simulink model "sensorExpoler_Lab1_4"  (R2026a)
settings: Solver=FixedStepDiscrete  StopTime=inf  FixedStep=0.001
undefined symbols (not defined in the file or in its folder): Blocking, Non
libraries: amg_usbconverter_n_connect_lib x2
settings Model: Creator=pboon  LastModifiedBy=supha

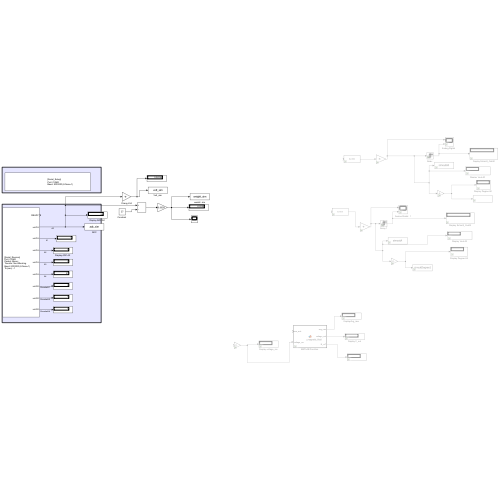
[thumbnail: Simulink's stored preview of the top-level diagram]
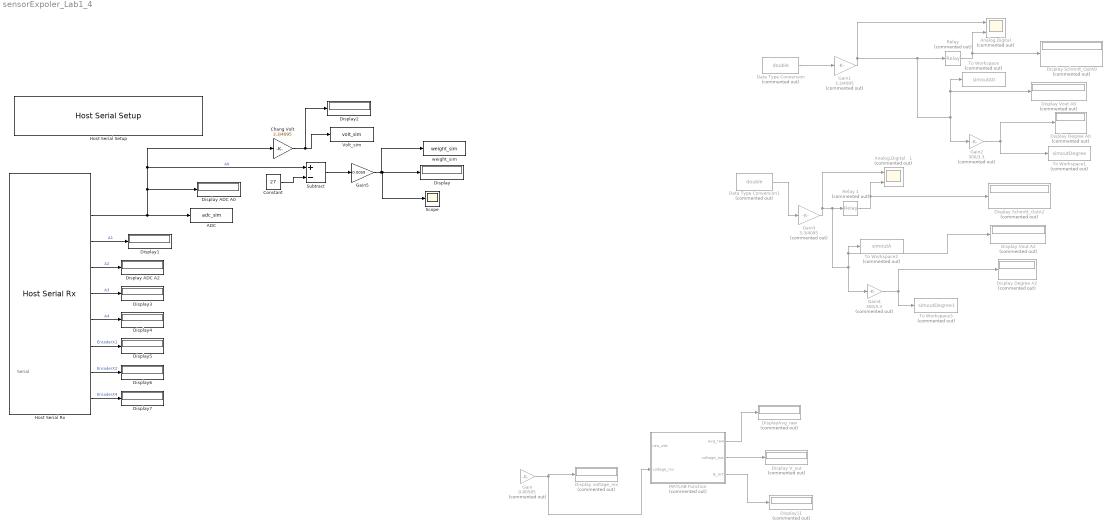
== system sensorExpoler_Lab1_4 ==
  note: Serial
  ADC : ToWorkspace  VariableName=adc_sim  SampleTime=-1
  "Analog,Digital   " : Scope  Commented=on  NumInputPorts=2
      settings: ActiveDisplayYMinimum=-0.17749084249084246  ActiveDisplayYMaximum=1.5974175824175825
  Analog,Digital   1 : Scope  Commented=on  NumInputPorts=2
      settings: ActiveDisplayYMinimum=-0.1684249084249084  ActiveDisplayYMaximum=1.5158241758241759
  Chang Volt : Gain  Gain=3.3/4095
  "Constant " : Constant  Value=27
  Data Type Conversion : DataTypeConversion  Commented=on  OutDataTypeStr=double  SaturateOnIntegerOverflow=off  RndMeth=Floor
  Data Type Conversion1 : DataTypeConversion  Commented=on  OutDataTypeStr=double  SaturateOnIntegerOverflow=off  RndMeth=Floor
  Display{,1..7} (8 alike) : Display
  "Display ADC A0 " : Display
  "Display ADC A2 " : Display
  "Display Degree A0 " : Display  Commented=on
  Display Degree A2 : Display  Commented=on
  Display Schmitt_OutA0 : Display  Commented=on
  Display Schmitt_OutA2 : Display  Commented=on
  "Display V_out " : Display  Commented=on
  "Display Vout A0 " : Display  Commented=on
  Display Vout A2 : Display  Commented=on
  "Display voltage_mv " : Display  Commented=on
  Display11 : Display  Commented=on
  "DisplayAvg_raw " : Display  Commented=on
  Gain : Gain  Commented=on  Gain=0.80585
  Gain1 : Gain  Commented=on  Gain=3.3/4095
  Gain2 : Gain  Commented=on  Gain=300/3.3
  Gain3 : Gain  Commented=on  Gain=3.3/4095
  Gain4 : Gain  Commented=on  Gain=300/3.3
  Gain5 : Gain  Gain=0.0059
  Host Serial Rx : amg_usbconverter_n_connect_lib/Host Serial Rx  conf=rx  port=<auto>  baudrate=2000000  databits=8  parity=None  stopbit=1  flowcontrol=None  transfer=Non-Blocking  timeout=5  packetmode=Binary  enableinitialvalues=off  initialvalues=[]  binheader='25'  binterminator='4E 4E'  porttype_double=0  porttype_single=0  porttype_int8=0  porttype_uint8=0  porttype_int16=0  porttype_uint16=5  porttype_int32=0  porttype_uint32=3  asciiformat='%d,%f'  rx_asciiterminator="CRLF (0x0D 0x0A - \"\\r\\n\")"  tx_asciiterminator="CRLF (0x0D 0x0A - \"\\r\\n\")"  sampletime=0.001  enablecustomportlabel=off  cinputportlabel=0  coutputportlabel=A  portpinstr=0  blockid=HostSerialRx  inputporttype=[]  inputportwidth=[]  inputportlabel={}  outputporttype=[3 5 5 5 5 5 7 7 7]  outputportwidth=[1 1 1 1 1 1 1 1 1]  outputportlabel={'READY','uint16','uint16','uint16','uint16','uint16','uint32','uint32','uint32'}  compat=0  optionstring=[]  autoport='COM4'
  Host Serial Setup : amg_usbconverter_n_connect_lib/Host Serial Setup  conf=setup  port=<auto>  baudrate=2000000  databits=8  parity=None  stopbit=1  flowcontrol=None  transfer=Blocking  timeout=2  packetmode=Binary  initialvalues=[]  binheader='7E 7E'  binterminator='03 03'  porttype_double=0  porttype_single=1  porttype_int8=0  porttype_uint8=0  porttype_int16=0  porttype_uint16=0  porttype_int32=0  porttype_uint32=2  asciiformat='%d %u %x'  rx_asciiterminator="CRLF (0x0D 0x0A - \"\\r\\n\")"  tx_asciiterminator="CRLF (0x0D 0x0A - \"\\r\\n\")"  sampletime=-1  enablecustomportlabel=off  cinputportlabel=0  coutputportlabel=A  portpinstr=0  blockid=HostSerialSetup  inputporttype=[]  inputportwidth=[]  inputportlabel={}  outputporttype=[]  outputportwidth=[]  outputportlabel={}  compat=0  optionstring=[]  autoport='COM4'
  "MATLAB Function " : MATLAB Function  Commented=on  TreatAsAtomicUnit=on
  "Relay " : Relay  Commented=on  OnSwitchValue=2.2  OffSwitchValue=1.1
  Relay 1 : Relay  Commented=on  OnSwitchValue=2.2  OffSwitchValue=1.1
  Scope : Scope
      settings: ActiveDisplayYMinimum=-1  ActiveDisplayYMaximum=1  DataLoggingVariableName=ScopeData2
  Subtract : Sum  Inputs=+-
  To Workspace : ToWorkspace  Commented=on  VariableName=simoutA0  SaveFormat=Timeseries  SampleTime=-1
  To Workspace1 : ToWorkspace  Commented=on  VariableName=simoutDegree  SaveFormat=Timeseries  SampleTime=-1
  To Workspace2 : ToWorkspace  Commented=on  VariableName=simoutA  SaveFormat=Timeseries  SampleTime=-1
  To Workspace3 : ToWorkspace  Commented=on  VariableName=simoutDegree1  SaveFormat=Timeseries  SampleTime=-1
  Volt_sim : ToWorkspace  VariableName=volt_sim  SampleTime=-1
  weight_sim : ToWorkspace  VariableName=weight_sim  SampleTime=-1
  wires:
  Host Serial Rx/2 -> Subtract/1, Chang Volt/1, "Display ADC A0 "/1, ADC/1  "A0"
  Host Serial Rx/3 -> Display1/1  "A1"
  Host Serial Rx/4 -> "Display ADC A2 "/1  "A2"
  Host Serial Rx/5 -> Display3/1  "A3"
  Host Serial Rx/6 -> Display4/1  "A4"
  Host Serial Rx/7 -> Display5/1  "EncoderX1"
  Host Serial Rx/8 -> Display6/1  "EncoderX2"
  Host Serial Rx/9 -> Display7/1  "EncoderX4"
  Gain/1 -> "Display voltage_mv "/1, "MATLAB Function "/2(voltage_mv)
  "MATLAB Function "/1(avg_raw) -> "DisplayAvg_raw "/1
  "MATLAB Function "/2(voltage_out) -> "Display V_out "/1
  "MATLAB Function "/3(B_mT) -> Display11/1
  Data Type Conversion/1 -> Gain1/1
  Gain1/1 -> "Analog,Digital   "/1, "Relay "/1, To Workspace/1, "Display Vout A0 "/1, Gain2/1
  "Relay "/1 -> "Analog,Digital   "/2, Display Schmitt_OutA0/1
  Gain2/1 -> To Workspace1/1, "Display Degree A0 "/1
  Gain4/1 -> To Workspace3/1, Display Degree A2/1
  Data Type Conversion1/1 -> Gain3/1
  Relay 1/1 -> Analog,Digital   1/2, Display Schmitt_OutA2/1
  Gain3/1 -> Analog,Digital   1/1, Relay 1/1, To Workspace2/1, Display Vout A2/1, Gain4/1
  Gain5/1 -> weight_sim/1, Scope/1, Display/1
  Subtract/1 -> Gain5/1
  "Constant "/1 -> Subtract/2
  Chang Volt/1 -> Display2/1, Volt_sim/1

== matlab function sensorExpoler_Lab1_4/MATLAB Function  ==
  data: raw_adc input; avg_raw output; voltage_out output; B_mT output; voltage_mv input
function [avg_raw, voltage_out, B_mT] = calculate_magnetic_field(raw_adc, voltage_mv)

% 1. ส่งค่า Raw ADC ออกไปโชว์ที่ Display
avg_raw = double(raw_adc);

% 2. ส่งค่าแรงดันไฟฟ้าที่รับมาจาก Gain ด้านนอก ออกไปโชว์ที่ Display
voltage_out = voltage_mv;

% 3. คำนวณความเข้มสนามแม่เหล็ก (B) จากค่า voltage_mv ที่รับเข้ามาจากพอร์ตซ้ายล่าง
VQ = 1650.0;          % แรงดันพัก (mV) ขณะไม่มีแม่เหล็ก
Sensitivity = 30.0;   % ค่าความไวเซนเซอร์ (mV/mT)

B_mT = (voltage_mv - VQ) / Sensitivity;

end
